simulink model "SILexample"  (R2024a)
settings: Solver=ode8  StartTime=0.0  StopTime=inf  FixedStep=SampleTime  RelTol=1e-3
undefined symbols (not defined in the file or in its folder): Arm, CDDrone, CDval, contact, control, ddx, ddy, ddz, dx, dy, dz, fractalcoef, g, lastVh, m, m_to_mm, p, pitch, prop_inertia, q, R, r, ref_height, ref_lat, ref_lon, roll, rotorRPMMax, rotorTimeConst, SampleTime, tilt_speed, X, Y, yaw, Z
libraries: sharedutil x3, robotcorelib x2, simulink x2, library_GPSPackaging x1, library_IMUPackaging x1, library_PX4SITLSFunc x1, shared6dof x1, simulink_extras x1, matrix_library x1, aerolibatmos2 x1, sensorgpslib x1, mspsensorlib x1
(part 1 of 2)
settings Model: Creator=tommy  LastModifiedBy=tommy

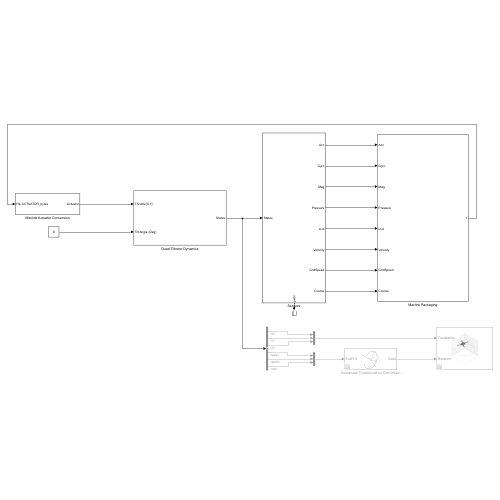
[thumbnail: Simulink's stored preview of the top-level diagram]
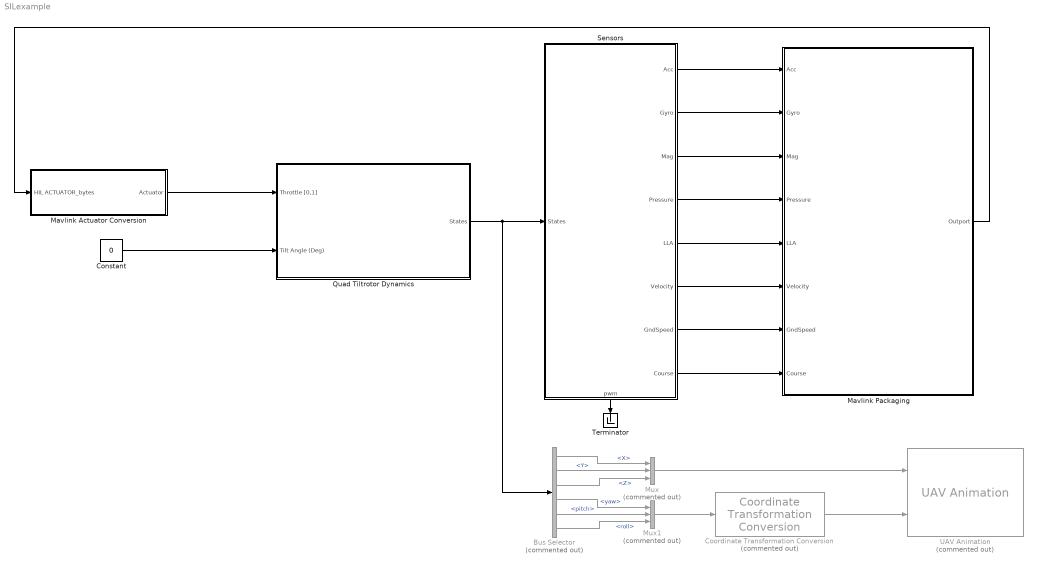
== system SILexample ==
  Bus Selector : BusSelector  Commented=on  OutputSignals=X,Y,Z,yaw,pitch,roll
  Constant : Constant  Value=0
  Coordinate Transformation Conversion : robotcorelib/Coordinate Transformation Conversion  Commented=on  InputRepresentation=Euler Angles  InputEulerSequence=ZYX  ShowTrVecInputPort=on  OutputRepresentation=Quaternion  OutputEulerSequence=ZYX  ShowTrVecOutputPort=on  SimulateUsing=Code generation
      settings: LibrarySourceBlock=uavutilslib/Coordinate Transformation Conversion
  Mavlink Actuator Conversion : Subsystem
  Mavlink Packaging : Subsystem
  Mux : Mux  Commented=on  Inputs=3
  Mux1 : Mux  Commented=on  Inputs=3
  Quad Tiltrotor Dynamics : Subsystem
  Sensors : Subsystem
      settings: PortSchema="{\"entries\":[{\"content\":{\"sides\":[{\"content\":{\"connectorIds\":[\"In1\"]},\"type\":\"ConnectorPlacement.EquallySpacedRectSide\",\"uuid\":\"4002fad5-cd2c-424c-b237-bc5c8c05716b\"},{\"content\":{\"connectorIds\":[\"Out1\",\"Out2\",\"Out3\",\"Out4\",\"Out5\",\"Out6\",\"Out7\",\"Out8\"],\"side\":\"RIGHT\"},\"type\":\"ConnectorPlacement.EquallySpacedRectSide\",\"uuid\":\"9eebcde2-0965-4c2d-bc23-958f112ae05f\"},{\"content\":{\"side\":\"TOP\"},\"type\":\"ConnectorPlacement.EquallySpacedRectSide\",\"uuid\":\"9f4a4643-69fe-47ac-ba33-df4cff119766\"},{\"content\":{\"connectorIds\":[\"Out9\"],\"side\":\"BOTTOM\"},\"type\":\"ConnectorPlacement.EquallySpacedRectSide\",\"uuid\":\"695c39dd-b607-453f-b052-38e279c7d42a\"}]},\"type\":\"ConnectorPlacement.EquallySpacedConnector\",\"uuid\":\"5d7ecaa3-fdec-470f-a1e1-b10a07dfac93\"}],\"packageUris\":[\"http://schema.mathworks.com/mf0/Connector/R2020b\"],\"version\":\"1.0\"}"
  Terminator : Terminator
  UAV Animation : uavutilslib/UAV Animation  Commented=on  UAVType=Multirotor  UAVSize=1  InertialZDirection=Down  SampleTime=0.04
  wires:
  Sensors/5(LLA) -> Mavlink Packaging/5(LLA)
  Sensors/1(Acc) -> Mavlink Packaging/1(Acc)
  Sensors/2(Gyro) -> Mavlink Packaging/2(Gyro)
  Sensors/3(Mag) -> Mavlink Packaging/3(Mag)
  Sensors/4(Pressure) -> Mavlink Packaging/4(Pressure)
  Sensors/6(Velocity) -> Mavlink Packaging/6(Velocity)
  Sensors/7(GndSpeed) -> Mavlink Packaging/7(GndSpeed)
  Sensors/8(Course) -> Mavlink Packaging/8(Course)
  Quad Tiltrotor Dynamics/1(States) -> Bus Selector/1, Sensors/1(States)
  Mavlink Actuator Conversion/1(Actuator) -> Quad Tiltrotor Dynamics/1(Throttle [0,1])
  Constant/1 -> Quad Tiltrotor Dynamics/2(Tilt Angle (Deg))
  Mux/1 -> UAV Animation/1
  Mux1/1 -> Coordinate Transformation Conversion/1
  Bus Selector/1 -> Mux/1  "<X>"
  Bus Selector/2 -> Mux/2  "<Y>"
  Bus Selector/3 -> Mux/3  "<Z>"
  Coordinate Transformation Conversion/1 -> UAV Animation/2
  Bus Selector/4 -> Mux1/1  "<yaw>"
  Bus Selector/5 -> Mux1/2  "<pitch>"
  Bus Selector/6 -> Mux1/3  "<roll>"
  Sensors/9(pwm) -> Terminator/1
  Mavlink Packaging/1(Outport) -> Mavlink Actuator Conversion/1(HIL ACTUATOR_bytes)

== system SILexample/Mavlink Actuator Conversion ==
  HIL ACTUATOR_bytes : Inport
  Data Type Conversion : DataTypeConversion  OutDataTypeStr=double  SaturateOnIntegerOverflow=off  RndMeth=Floor
  Rate Transition : RateTransition  OutPortSampleTime=SampleTime
  Saturation : Saturate  UpperLimit=1  LowerLimit=0
  Selector1 : Selector  InputPortWidth=16  IndexOptions=Index vector (dialog)  Indices=[1:4]  OutputSizes=1
  Actuator : Outport
  wires:
  Saturation/1 -> Actuator/1
  Data Type Conversion/1 -> Selector1/1
  Selector1/1 -> Saturation/1  "Controls"
  HIL ACTUATOR_bytes/1 -> Rate Transition/1
  Rate Transition/1 -> Data Type Conversion/1

== system SILexample/Mavlink Packaging ==
  Acc : Inport
  Gyro : Inport  Port=2
  Mag : Inport  Port=3
  Pressure : Inport  Port=4
  LLA : Inport  Port=5
  Velocity : Inport  Port=6
  GndSpeed : Inport  Port=7
  Course : Inport  Port=8
  GPSPackaging : library_GPSPackaging/GPSPackaging
  IMUPackaging : library_IMUPackaging/IMUPackaging
  PX4SITLSFunc : library_PX4SITLSFunc/PX4SITLSFunc
  Outport : Outport
  wires:
  Acc/1 -> IMUPackaging/1
  PX4SITLSFunc/1 -> Outport/1
  IMUPackaging/1 -> PX4SITLSFunc/1
  Gyro/1 -> IMUPackaging/2
  Mag/1 -> IMUPackaging/3
  Pressure/1 -> IMUPackaging/4
  LLA/1 -> GPSPackaging/1
  Velocity/1 -> GPSPackaging/2
  GndSpeed/1 -> GPSPackaging/3
  Course/1 -> GPSPackaging/4
  GPSPackaging/1 -> PX4SITLSFunc/2

== system SILexample/Quad Tiltrotor Dynamics ==
  note: Goals for this model : A novel vortex ring state escape mechanism for a quad tilt-rotor vehicle.
      |
      | 1. accurately portray thrust forces in a quad-tilt rotor vehicle in an in-place descent to design a controller for
      | - curve fits from CFD for descent in both non tilted and tilted configurations
      |
      | 2. simple transition model since horizontal forces and torques cancel out in both configurations
      | - transition interpolates forces between non tilted and tilted curves (based on angle)
      |
      | 3. simple model for torques since this research focuses more on in-place descents and less on attitude control
      | - torque model based on simple aerodynamics, e.g., assumption of constant Cd
  note: Note:
      |
      | DCM_be converts a vector written in earth frame to body frame
      | Abe is acceleration of body written in body frame, but measured relative to earth.
      | To get acceleration of body written in earth frame (NED fixed on takeoff location), we need to convert the frame.
      | IMU block's angular velocity and acceleration inputs are written in earth frame (NED)
  Throttle [0,1] : Inport
  Tilt Angle (Deg) : Inport  Port=2
  6DOF (Quaternion) : shared6dof/6DOF (Euler Angles)  units=Metric (MKS)  mtype=Fixed  rep=Quaternion  xme_0=init.posNED  Vm_0=init.vb  eul_0=init.euler  pm_0=init.angRates  mass_0=m  mass_e=0.5  mass_f=2.0  inertia=inertia  inertia_e=eye(3)  inertia_f=2*eye(3)  k_quat=1  vre_flag=on  abi_flag=on  aMode=0  xme_statename=''  Vm_statename=''  eul_statename=''  quat_statename=''  pm_statename=''  mass_statename=''
      settings: LibrarySourceBlock=aerolib6dof2/6DOF (Quaternion)
  Airframe : Subsystem
      mask Display: image('PX4-Quad-X-Motor-Configuration-33.png', [5,0,0,0,80,50]);
  Motor Model : Subsystem
  Rate Transition : RateTransition  OutPortSampleTime=SampleTime
  States Bus : Subsystem
  Terminator : Terminator
  Terminator1 : Terminator
  States : Outport
  wires:
  States Bus/1(States) -> Rate Transition/1
  Rate Transition/1 -> States/1
  6DOF (Quaternion)/7 -> Terminator/1
  6DOF (Quaternion)/4 -> Airframe/4(DCMbe), States Bus/4(DCMbe)
  6DOF (Quaternion)/6 -> Airframe/6(Wb), States Bus/5(Wb)
  Airframe/1(F_cg) -> 6DOF (Quaternion)/1
  6DOF (Quaternion)/2 -> States Bus/2(Xe), Airframe/5(Xe)
  Airframe/2(M_cg) -> 6DOF (Quaternion)/2
  6DOF (Quaternion)/9 -> States Bus/6(acc_lnav)
  6DOF (Quaternion)/5 -> Airframe/3(Vb)
  6DOF (Quaternion)/8 -> Terminator1/1
  6DOF (Quaternion)/3 -> Airframe/7(rpy), States Bus/3(rpy)
  6DOF (Quaternion)/1 -> States Bus/1(Ve)
  Tilt Angle (Deg)/1 -> Airframe/2(Tilt Angle (Deg))
  Throttle [0,1]/1 -> Motor Model/1(Throttle)
  Motor Model/1(RPM) -> Airframe/1(rpm)

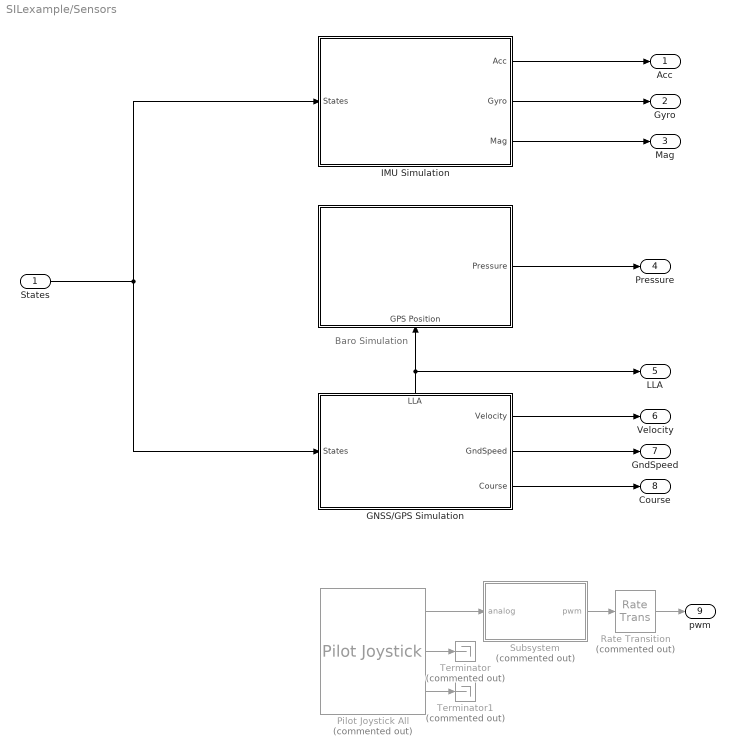
== system SILexample/Sensors ==
  note: Baro Simulation
  States : Inport
  " " : Subsystem
      settings: PortSchema="{\"entries\":[{\"content\":{\"sides\":[{\"content\":{\"connectorIds\":[]},\"type\":\"ConnectorPlacement.EquallySpacedRectSide\",\"uuid\":\"7ecc8b21-8f8f-4144-826a-6b68e30dbf7d\"},{\"content\":{\"connectorIds\":[\"Out1\"],\"side\":\"RIGHT\"},\"type\":\"ConnectorPlacement.EquallySpacedRectSide\",\"uuid\":\"81a1dd55-8330-4386-9921-36c0eb60d526\"},{\"content\":{\"connectorIds\":[],\"side\":\"TOP\"},\"type\":\"ConnectorPlacement.EquallySpacedRectSide\",\"uuid\":\"b99caff5-b40d-407d-b30e-35210c1aee1d\"},{\"content\":{\"connectorIds\":[\"In1\"],\"side\":\"BOTTOM\"},\"type\":\"ConnectorPlacement.EquallySpacedRectSide\",\"uuid\":\"18bfda3d-4fab-4e61-9ebc-e384e51de306\"}]},\"type\":\"ConnectorPlacement.EquallySpacedConnector\",\"uuid\":\"17ab4e96-b761-4c62-a0bb-ab626dac3eaa\"}],\"packageUris\":[\"http://schema.mathworks.com/mf0/Connector/R2020b\"],\"version\":\"1.0\"}"
  GNSS/GPS Simulation : Subsystem
      settings: PortSchema="{\"entries\":[{\"content\":{\"sides\":[{\"content\":{\"connectorIds\":[\"In1\"]},\"type\":\"ConnectorPlacement.EquallySpacedRectSide\",\"uuid\":\"4934e8ff-5d4b-4e11-968d-c23bd62383a0\"},{\"content\":{\"connectorIds\":[\"Out1\",\"Out2\",\"Out3\"],\"side\":\"RIGHT\"},\"type\":\"ConnectorPlacement.EquallySpacedRectSide\",\"uuid\":\"9ec8bc0a-2d3c-4dca-835c-010ac29b6ebc\"},{\"content\":{\"connectorIds\":[\"Out4\"],\"side\":\"TOP\"},\"type\":\"ConnectorPlacement.EquallySpacedRectSide\",\"uuid\":\"04f09eb4-1bd9-450e-b951-47054bdd92ad\"}]},\"type\":\"ConnectorPlacement.EquallySpacedConnector\",\"uuid\":\"9a5920cf-a58d-4c98-839b-fbac94edbe7e\"}],\"packageUris\":[\"http://schema.mathworks.com/mf0/Connector/R2020b\"],\"version\":\"1.0\"}"
  IMU Simulation : Subsystem
  Pilot Joystick All : aerolibanimutils/Pilot Joystick  Commented=on  JoystickID=Joystick1  OutputConfiguration=AllOutputs  SampleTime=0.04
  Rate Transition : RateTransition  Commented=on  OutPortSampleTime=SampleTime
  Subsystem : Subsystem  Commented=on
  Terminator : Terminator  Commented=on
  Terminator1 : Terminator  Commented=on
  Acc : Outport
  Gyro : Outport  Port=2
  Mag : Outport  Port=3
  Pressure : Outport  Port=4
  LLA : Outport  Port=5
  Velocity : Outport  Port=6
  GndSpeed : Outport  Port=7
  Course : Outport  Port=8
  pwm : Outport  Port=9
  wires:
  IMU Simulation/3(Mag) -> Mag/1
  GNSS/GPS Simulation/4(LLA) -> LLA/1, " "/1(GPS Position)
  GNSS/GPS Simulation/2(GndSpeed) -> GndSpeed/1
  States/1 -> GNSS/GPS Simulation/1(States), IMU Simulation/1(States)
  IMU Simulation/2(Gyro) -> Gyro/1
  IMU Simulation/1(Acc) -> Acc/1
  GNSS/GPS Simulation/1(Velocity) -> Velocity/1
  GNSS/GPS Simulation/3(Course) -> Course/1
  " "/1(Pressure) -> Pressure/1
  Pilot Joystick All/1 -> Subsystem/1(analog)
  Pilot Joystick All/2 -> Terminator/1
  Pilot Joystick All/3 -> Terminator1/1
  Subsystem/1(pwm) -> Rate Transition/1
  Rate Transition/1 -> pwm/1

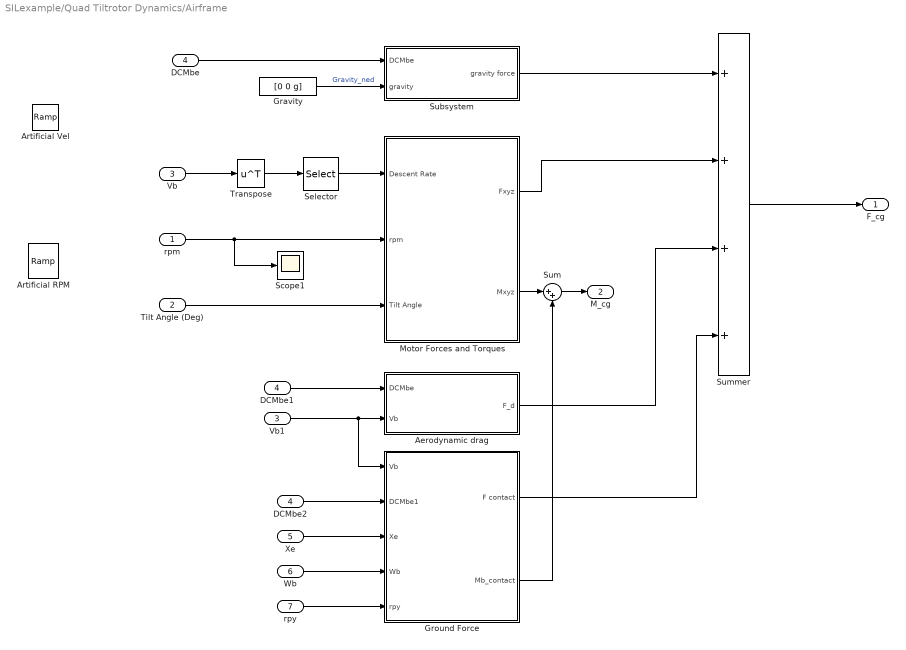
== system SILexample/Quad Tiltrotor Dynamics/Airframe ==
  rpm : Inport
  Tilt Angle (Deg) : Inport  Port=2
  Vb : Inport  Port=3
  DCMbe : Inport  Port=4
  Xe : Inport  Port=5
  Wb : Inport  Port=6
  rpy : Inport  Port=7
  Aerodynamic drag : Subsystem
  Artificial RPM : simulink/Sources/Ramp  slope=[0;-0;0;-0]  start=0  InitialOutput=[-3000; 3000; -2000; 2000]  VectorParams1D=off
  Artificial Vel : simulink/Sources/Ramp  slope=[0;0;0]  start=0  InitialOutput=[0;0;0]  VectorParams1D=off
  DCMbe1 : InportShadow  Port=4
  DCMbe2 : InportShadow  Port=4
  Gravity : Constant  Value=[0 0 g]
  Ground Force : Subsystem
  Motor Forces and Torques : Subsystem
  Scope1 : Scope
  Selector : Selector  InputPortWidth=3  IndexOptions=Index vector (dialog)  Indices=[3]  OutputSizes=1
  Subsystem : Subsystem
  Sum : Sum  Inputs=|++
  Summer : Sum  Inputs=++++
  Transpose : Math  Operator=transpose
  Vb1 : InportShadow  Port=3
  F_cg : Outport
  M_cg : Outport  Port=2
  wires:
  Subsystem/1(gravity force) -> Summer/1
  rpm/1 -> Scope1/1, Motor Forces and Torques/2(rpm)
  Motor Forces and Torques/1(Fxyz) -> Summer/2
  Gravity/1 -> Subsystem/2(gravity)  "Gravity_ned"
  DCMbe/1 -> Subsystem/1(DCMbe)
  Transpose/1 -> Selector/1
  Selector/1 -> Motor Forces and Torques/1(Descent Rate)
  Tilt Angle (Deg)/1 -> Motor Forces and Torques/3(Tilt Angle)
  Summer/1 -> F_cg/1
  Vb/1 -> Transpose/1
  DCMbe2/1 -> Ground Force/2(DCMbe1)
  Vb1/1 -> Ground Force/1(Vb), Aerodynamic drag/2(Vb)
  Xe/1 -> Ground Force/3(Xe)
  Aerodynamic drag/1(F_d) -> Summer/3
  Ground Force/1(F contact) -> Summer/4
  Ground Force/2(Mb_contact) -> Sum/2
  Motor Forces and Torques/2(Mxyz) -> Sum/1
  Sum/1 -> M_cg/1
  rpy/1 -> Ground Force/5(rpy)
  Wb/1 -> Ground Force/4(Wb)
  DCMbe1/1 -> Aerodynamic drag/1(DCMbe)

== system SILexample/Quad Tiltrotor Dynamics/Motor Model ==
  Throttle : Inport
  Demux : Demux
  Gain : Gain  Gain=[-1;-1;1;1]
  Mux : Mux
  Transfer Fcn{,2..4} (4 alike) : TransferFcn  Numerator=[rotorRPMMax]  Denominator=[rotorTimeConst 1]
  RPM : Outport
  wires:
  Mux/1 -> Gain/1
  Transfer Fcn/1 -> Mux/4
  Demux/4 -> Transfer Fcn/1
  Transfer Fcn3/1 -> Mux/2
  Transfer Fcn2/1 -> Mux/3
  Demux/1 -> Transfer Fcn4/1
  Demux/3 -> Transfer Fcn2/1
  Demux/2 -> Transfer Fcn3/1
  Transfer Fcn4/1 -> Mux/1
  Gain/1 -> RPM/1
  Throttle/1 -> Demux/1

== system SILexample/Quad Tiltrotor Dynamics/States Bus ==
  Ve : Inport
  Xe : Inport  Port=2
  rpy : Inport  Port=3
  DCMbe : Inport  Port=4
  Wb : Inport  Port=5
  acc_lnav : Inport  Port=6
  Bus Creator : BusCreator  Inputs=X,Y,Z,yaw,pitch,roll,dx,dy,dz,p,q,r,ddx,ddy,ddz
  Demux{,1..4} (5 alike) : Demux  Outputs=3
  Matrix Multiply : Product  Multiplication=Matrix(*)
  Matrix Multiply1 : Product  Multiplication=Matrix(*)
  Transpose : Math  Operator=transpose
  ypr : Selector  InputPortWidth=3  IndexOptions=Index vector (dialog)  Indices=[3 2 1]  OutputSizes=1
  States : Outport
  wires:
  Demux1/1 -> Bus Creator/1  "X"
  Demux1/2 -> Bus Creator/2  "Y"
  rpy/1 -> ypr/1
  Demux2/2 -> Bus Creator/5  "pitch"
  Demux3/2 -> Bus Creator/8  "dy"
  Demux2/3 -> Bus Creator/6  "roll"
  Ve/1 -> Demux3/1
  Demux2/1 -> Bus Creator/4  "yaw"
  Demux1/3 -> Bus Creator/3  "Z"
  Demux3/1 -> Bus Creator/7  "dx"
  Demux4/2 -> Bus Creator/11  "q"
  Demux3/3 -> Bus Creator/9  "dz"
  Demux4/3 -> Bus Creator/12  "r"
  Demux4/1 -> Bus Creator/10  "p"
  Bus Creator/1 -> States/1
  Xe/1 -> Demux1/1
  Demux/3 -> Bus Creator/15  "ddz"
  Demux/2 -> Bus Creator/14  "ddy"
  Demux/1 -> Bus Creator/13  "ddx"
  Matrix Multiply/1 -> Demux4/1
  DCMbe/1 -> Transpose/1
  Transpose/1 -> Matrix Multiply1/1, Matrix Multiply/1
  Wb/1 -> Matrix Multiply/2
  acc_lnav/1 -> Matrix Multiply1/2
  Matrix Multiply1/1 -> Demux/1
  ypr/1 -> Demux2/1

== system SILexample/Sensors/  ==
  GPS Position : Inport
  Extract Altitude : Selector  InputPortWidth=3  IndexOptions=Index vector (dialog)  Indices=[3]  OutputSizes=1
  Gain1 : Gain  Gain=1/m_to_mm
  Gain2 : Gain  Gain=m_to_mm
  Lapse Rate Model : aerolibatmos2/ISA Atmosphere Model  useExtended=off  action=Warning  custom=on  viscosityOut=off  g=9.80665  gamma=1.4  R=287.0531  L=0.0065  h_trop=11000  h_strat=20000  rho0=1.225  P0=101325  T0=288.15  h0=0  S=110.4  Tref=273.15  muref=1.716e-5
  Random Number1 : RandomNumber  Variance=10000  Seed=10  SampleTime=SampleTime
  Sum1 : Sum  Inputs=|++
  Terminator : Terminator
  Terminator1 : Terminator
  Terminator2 : Terminator
  Pressure : Outport
  wires:
  Lapse Rate Model/2 -> Terminator1/1
  Lapse Rate Model/4 -> Terminator2/1
  Lapse Rate Model/1 -> Terminator/1
  Lapse Rate Model/3 -> Pressure/1
  Sum1/1 -> Gain1/1
  Gain2/1 -> Sum1/1
  Extract Altitude/1 -> Gain2/1
  Gain1/1 -> Lapse Rate Model/1
  GPS Position/1 -> Extract Altitude/1
  Random Number1/1 -> Sum1/2  "Pressure_noise"

== system SILexample/Sensors/GNSS//GPS Simulation ==
  States : Inport
  Bus Selector : BusSelector  OutputSignals=dx,dy,dz  OutputAsBus=on
  Bus Selector1 : BusSelector  OutputSignals=X,Y,Z  OutputAsBus=on
  GPS : sensorgpslib/GPS  DispRefFrame=NED  PositionInputFormat=Local  ReferenceLocation=[ref_lat ref_lon ref_height]  HorizontalPositionAccuracy=0.01  VerticalPositionAccuracy=0.01  VelocityAccuracy=0.01  DecayFactor=0.99  SeedDouble=67  SimulateUsing=Interpreted execution
  Reshape1 : Reshape  OutputDimensionality=Row vector (2-D)
  Reshape3 : Reshape  OutputDimensionality=Row vector (2-D)
  Velocity : Outport
  GndSpeed : Outport  Port=2
  Course : Outport  Port=3
  LLA : Outport  Port=4
  wires:
  Reshape3/1 -> GPS/1
  GPS/1 -> LLA/1  "lla"
  Bus Selector1/1 -> Reshape3/1
  Bus Selector/1 -> Reshape1/1
  Reshape1/1 -> GPS/2
  GPS/2 -> Velocity/1
  States/1 -> Bus Selector/1, Bus Selector1/1
  GPS/3 -> GndSpeed/1
  GPS/4 -> Course/1

== system SILexample/Sensors/IMU Simulation ==
  note: Note:
      | we need accelerometer output)in A-G, but block outputs G-A.
  States : Inport
  Bus Selector1 : BusSelector  OutputSignals=p,q,r  OutputAsBus=on
  Bus Selector2 : BusSelector  OutputSignals=yaw,pitch,roll  OutputAsBus=on
  Bus Selector3 : BusSelector  OutputSignals=ddx,ddy,ddz  OutputAsBus=on
  Coordinate Transformation Conversion1 : robotcorelib/Coordinate Transformation Conversion  InputRepresentation=Euler Angles  InputEulerSequence=ZYX  ShowTrVecInputPort=on  OutputRepresentation=Quaternion  OutputEulerSequence=ZYX  ShowTrVecOutputPort=on  SimulateUsing=Interpreted execution
  Gain : Gain  Gain=-1
  IMU1 : mspsensorlib/IMU  DispRefFrame=NED  TemperaturePort=off  Temperature=25  MagneticFieldPort=off  MagneticFieldNED=[21.5 1.16 43.1]  MagneticFieldENU=[ -2.4169, 27.5550, 16.0849 ]  SeedDouble=87254  SimulateUsing=Interpreted execution  AccelParamsMeasurementRange=Inf  AccelParamsResolution=0  AccelParamsConstantBias=[ 0, 0, 0 ]  AccelParamsAxesMisalignment=[ 0, 0, 0 ]  AccelParamsNoiseDensity=0.0003  AccelParamsBiasInstability=[ 0, 0, 0 ]  AccelParamsBiasInstabilityNumerator=fractalcoef().Numerator  AccelParamsBiasInstabilityDenominator=fractalcoef().Denominator  AccelParamsRandomWalk=[ 0, 0, 0 ]  AccelParamsNoiseType=double-sided  AccelParamsTemperatureBias=[ 0, 0, 0 ]  AccelParamsTemperatureScaleFactor=[ 0, 0, 0 ]  GyroParamsMeasurementRange=Inf  GyroParamsResolution=0  GyroParamsConstantBias=[ 0, 0, 0 ]  GyroParamsAxesMisalignment=[ 0, 0, 0 ]  GyroParamsAccelerationBias=0.0001  GyroParamsNoiseDensity=0.01  GyroParamsBiasInstability=[ 0, 0, 0 ]  GyroParamsBiasInstabilityNumerator=fractalcoef().Numerator  GyroParamsBiasInstabilityDenominator=fractalcoef().Denominator  GyroParamsRandomWalk=[ 0, 0, 0 ]  GyroParamsNoiseType=double-sided  GyroParamsTemperatureBias=[ 0, 0, 0 ]  GyroParamsTemperatureScaleFactor=[ 0, 0, 0 ]  MagParamsMeasurementRange=Inf  MagParamsResolution=0  MagParamsConstantBias=[ 0, 0, 0 ]  MagParamsAxesMisalignment=[ 0, 0, 0 ]  MagParamsNoiseDensity=0.0001  MagParamsBiasInstability=[ 0, 0, 0 ]  MagParamsBiasInstabilityNumerator=fractalcoef().Numerator  MagParamsBiasInstabilityDenominator=fractalcoef().Denominator  MagParamsRandomWalk=[ 0, 0, 0 ]  MagParamsNoiseType=double-sided  MagParamsTemperatureBias=[ 0, 0, 0 ]  MagParamsTemperatureScaleFactor=[ 0, 0, 0 ]
  Reshape : Reshape  OutputDimensionality=Row vector (2-D)
  Reshape2 : Reshape  OutputDimensionality=Row vector (2-D)
  Reshape3 : Reshape  OutputDimensionality=Row vector (2-D)
  Acc : Outport
  Gyro : Outport  Port=2
  Mag : Outport  Port=3
  wires:
  Coordinate Transformation Conversion1/1 -> Reshape3/1
  Reshape3/1 -> IMU1/3
  IMU1/2 -> Gyro/1
  Reshape/1 -> IMU1/1
  Bus Selector3/1 -> Reshape/1
  IMU1/1 -> Gain/1
  Bus Selector1/1 -> Reshape2/1
  Bus Selector2/1 -> Coordinate Transformation Conversion1/1
  Reshape2/1 -> IMU1/2
  States/1 -> Bus Selector1/1, Bus Selector2/1, Bus Selector3/1
  Gain/1 -> Acc/1  "acc"
  IMU1/3 -> Mag/1

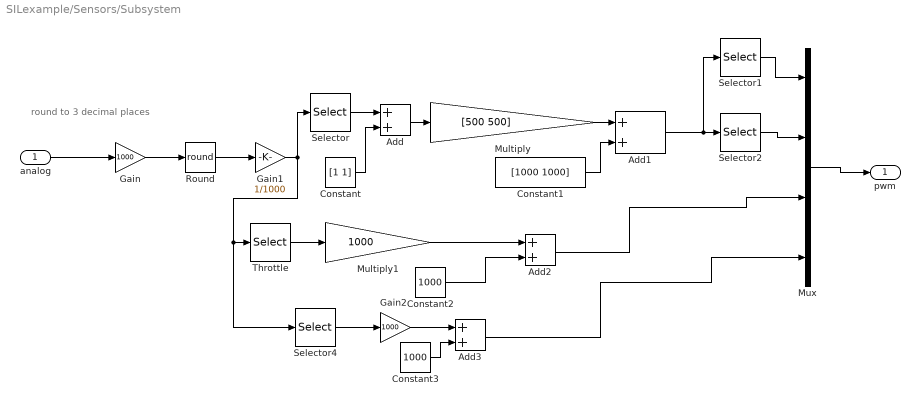
== system SILexample/Sensors/Subsystem ==
  note: round to 3 decimal places
  analog : Inport
  Add{,1..3} (4 alike) : Sum
  Constant : Constant  Value=[1 1]
  Constant1 : Constant  Value=[1000 1000]
  Constant2 : Constant  Value=1000
  Constant3 : Constant  Value=1000
  Gain : Gain  Gain=1000
  Gain1 : Gain  Gain=1/1000
  Gain2 : Gain  Gain=1000
  Multiply : Gain  Gain=[500 500]
  Multiply1 : Gain  Gain=1000
  Mux : Mux
  Round : Rounding  Operator=round
  Selector : Selector  InputPortWidth=6  IndexOptions=Index vector (dialog)  Indices=[1 2]  OutputSizes=1
  Selector1 : Selector  InputPortWidth=2  IndexOptions=Index vector (dialog)  Indices=[1]  OutputSizes=1
  Selector2 : Selector  InputPortWidth=2  IndexOptions=Index vector (dialog)  Indices=[2]  OutputSizes=1
  Selector4 : Selector  InputPortWidth=6  IndexOptions=Index vector (dialog)  Indices=[6]  OutputSizes=1
  Throttle : Selector  InputPortWidth=6  IndexOptions=Index vector (dialog)  Indices=[3]  OutputSizes=1
  pwm : Outport
  wires:
  Selector2/1 -> Mux/2
  Multiply/1 -> Add1/1
  Gain1/1 -> Selector4/1, Throttle/1, Selector/1
  Selector/1 -> Add/1
  Add1/1 -> Selector1/1, Selector2/1
  Gain/1 -> Round/1
  Constant/1 -> Add/2
  Constant2/1 -> Add2/2
  Add3/1 -> Mux/4
  Constant1/1 -> Add1/2
  Selector1/1 -> Mux/1
  analog/1 -> Gain/1
  Add/1 -> Multiply/1
  Round/1 -> Gain1/1
  Add2/1 -> Mux/3
  Throttle/1 -> Multiply1/1
  Multiply1/1 -> Add2/1
  Selector4/1 -> Gain2/1
  Constant3/1 -> Add3/2
  Gain2/1 -> Add3/1
  Mux/1 -> pwm/1

== system SILexample/Quad Tiltrotor Dynamics/Airframe/Aerodynamic drag ==
  DCMbe : Inport
  Vb : Inport  Port=2
  Add : Sum
  Constant : Constant  Value=[ 0 0 0]
  Constant1 : Constant  Value=CDDrone
  Display : Display
  Dot Product : DotProduct  OutDataTypeStr=Inherit: Inherit via internal rule
  Matrix Multiply : Product  Multiplication=Matrix(*)
  Product : Product  Inputs=3
  Saturation : Saturate  UpperLimit=inf  LowerLimit=0.0001
  Square Root : Sqrt
  gain : Gain  Gain=-1
  F_d : Outport
  wires:
  Saturation/1 -> Square Root/1
  Vb/1 -> gain/1
  Dot Product/1 -> Saturation/1
  Square Root/1 -> Product/1
  Constant1/1 -> Product/3
  DCMbe/1 -> Matrix Multiply/1
  Constant/1 -> Matrix Multiply/2
  gain/1 -> Add/2
  Matrix Multiply/1 -> Add/1
  Add/1 -> Dot Product/1, Dot Product/2, Product/2
  Product/1 -> Display/1, F_d/1

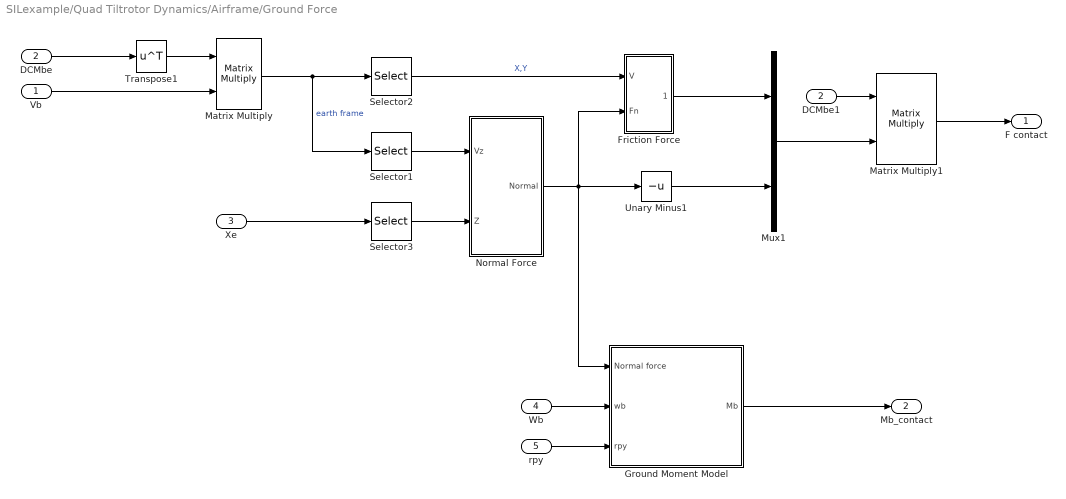
== system SILexample/Quad Tiltrotor Dynamics/Airframe/Ground Force ==
  Vb : Inport
  DCMbe1 : Inport  Port=2
  Xe : Inport  Port=3
  Wb : Inport  Port=4
  rpy : Inport  Port=5
  DCMbe : InportShadow  Port=2
  Friction Force : Subsystem
  Ground Moment Model : Subsystem
  Matrix Multiply : Product  Multiplication=Matrix(*)
  Matrix Multiply1 : Product  Multiplication=Matrix(*)
  Mux1 : Mux  Inputs=2
  Normal Force : Subsystem
  Selector1 : Selector  InputPortWidth=3  IndexOptions=Index vector (dialog)  Indices=[3]  OutputSizes=1
  Selector2 : Selector  InputPortWidth=3  IndexOptions=Index vector (dialog)  Indices=[1,2]  OutputSizes=1
  Selector3 : Selector  InputPortWidth=3  IndexOptions=Index vector (dialog)  Indices=[3]  OutputSizes=1
  Transpose1 : Math  Operator=transpose
  Unary Minus1 : UnaryMinus
  F contact : Outport
  Mb_contact : Outport  Port=2
  wires:
  Matrix Multiply1/1 -> F contact/1
  Friction Force/1(Friction) -> Mux1/1
  Xe/1 -> Selector3/1
  Vb/1 -> Matrix Multiply/2
  Selector3/1 -> Normal Force/2(Z)
  Matrix Multiply/1 -> Selector1/1, Selector2/1  "earth frame"
  Mux1/1 -> Matrix Multiply1/2
  Selector2/1 -> Friction Force/1(V)  "X,Y"
  Selector1/1 -> Normal Force/1(Vz)
  DCMbe1/1 -> Matrix Multiply1/1
  DCMbe/1 -> Transpose1/1
  Transpose1/1 -> Matrix Multiply/1
  Unary Minus1/1 -> Mux1/2
  Normal Force/1(Normal) -> Ground Moment Model/1(Normal force), Unary Minus1/1, Friction Force/2(Fn)
  Wb/1 -> Ground Moment Model/2(wb)
  rpy/1 -> Ground Moment Model/3(rpy)
  Ground Moment Model/1(Mb) -> Mb_contact/1

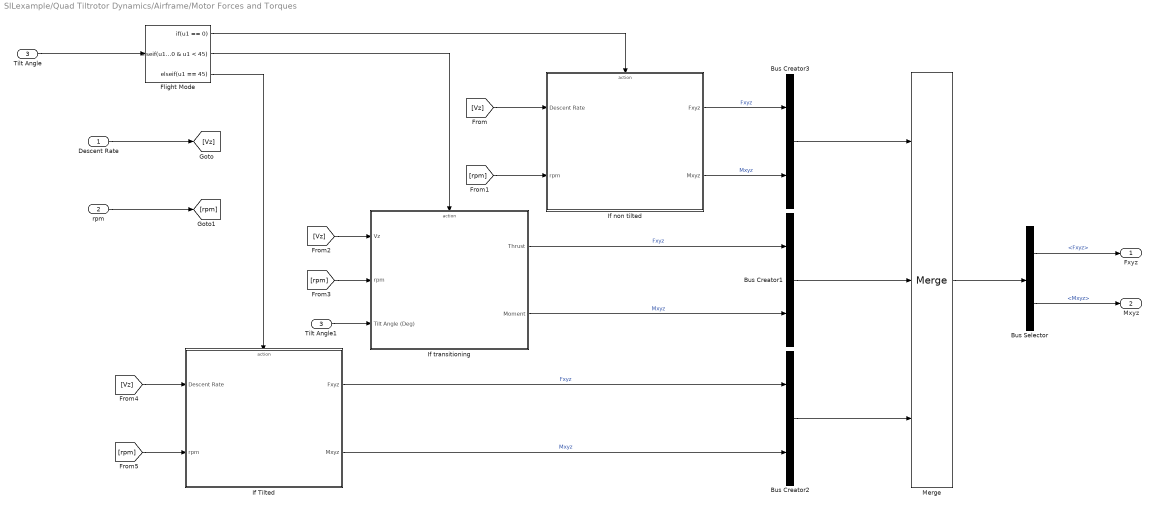
== system SILexample/Quad Tiltrotor Dynamics/Airframe/Motor Forces and Torques ==
  Descent Rate : Inport
  rpm : Inport  Port=2
  Tilt Angle : Inport  Port=3
  Bus Creator1 : BusCreator  Inputs=2
  Bus Creator2 : BusCreator  Inputs=2
  Bus Creator3 : BusCreator  Inputs=2
  Bus Selector : BusSelector  OutputSignals=Fxyz,Mxyz
  Flight Mode : If  IfExpression=u1 == 0  ElseIfExpressions=u1 > 0 & u1 < 45, u1 == 45  ShowElse=off
  If Tilted : Subsystem  TreatAsAtomicUnit=on
  If non tilted : Subsystem  TreatAsAtomicUnit=on
  If transitioning : Subsystem  TreatAsAtomicUnit=on
  Merge : Merge  Inputs=3  InitialOutput=[0]
  Tilt Angle1 : InportShadow  Port=3
  Fxyz : Outport
  Mxyz : Outport  Port=2
  wires:
  Flight Mode/3 -> If Tilted/Action
  Flight Mode/2 -> If transitioning/Action
  Flight Mode/1 -> If non tilted/Action
  Descent Rate/1 -> [Vz]
  rpm/1 -> [rpm]
  [Vz] -> If transitioning/1(Vz)
  [rpm] -> If transitioning/2(rpm)
  [Vz] -> If Tilted/1(Descent Rate)
  [rpm] -> If Tilted/2(rpm)
  If transitioning/1(Thrust) -> Bus Creator1/1  "Fxyz"
  If transitioning/2(Moment) -> Bus Creator1/2  "Mxyz"
  If Tilted/1(Fxyz) -> Bus Creator2/1  "Fxyz"
  If Tilted/2(Mxyz) -> Bus Creator2/2  "Mxyz"
  Bus Creator3/1 -> Merge/1
  Bus Creator1/1 -> Merge/2
  Merge/1 -> Bus Selector/1
  Bus Selector/1 -> Fxyz/1  "<Fxyz>"
  Bus Selector/2 -> Mxyz/1  "<Mxyz>"
  Bus Creator2/1 -> Merge/3
  If non tilted/1(Fxyz) -> Bus Creator3/1  "Fxyz"
  If non tilted/2(Mxyz) -> Bus Creator3/2  "Mxyz"
  [Vz] -> If non tilted/1(Descent Rate)
  [rpm] -> If non tilted/2(rpm)
  Tilt Angle1/1 -> If transitioning/3(Tilt Angle (Deg))
  Tilt Angle/1 -> Flight Mode/1

== system SILexample/Quad Tiltrotor Dynamics/Airframe/Subsystem ==
  DCMbe : Inport
  gravity : Inport  Port=2  Unit=m/s^2
  Gain1 : Gain  Gain=m
  Product : Product  Multiplication=Matrix(*)
  gravity force : Outport  Unit=N  VectorParamsAs1DForOutWhenUnconnected=off
  wires:
  gravity/1 -> Gain1/1
  Product/1 -> gravity force/1
  DCMbe/1 -> Product/1
  Gain1/1 -> Product/2  "gravity force NED"

== system SILexample/Quad Tiltrotor Dynamics/Airframe/Ground Force/Friction Force ==
  V : Inport
  Fn : Inport  Port=2
  Product : Product
  Saturation : Saturate  UpperLimit=contact.translation.maxFriction  LowerLimit=-contact.translation.maxFriction
  Soft Coulomb Friction : Subsystem
  Unary Minus : UnaryMinus
  Friction : Outport
  wires:
  Fn/1 -> Product/2
  Soft Coulomb Friction/1(Out1) -> Product/1
  Product/1 -> Unary Minus/1
  V/1 -> Soft Coulomb Friction/1(In1)
  Unary Minus/1 -> Saturation/1
  Saturation/1 -> Friction/1

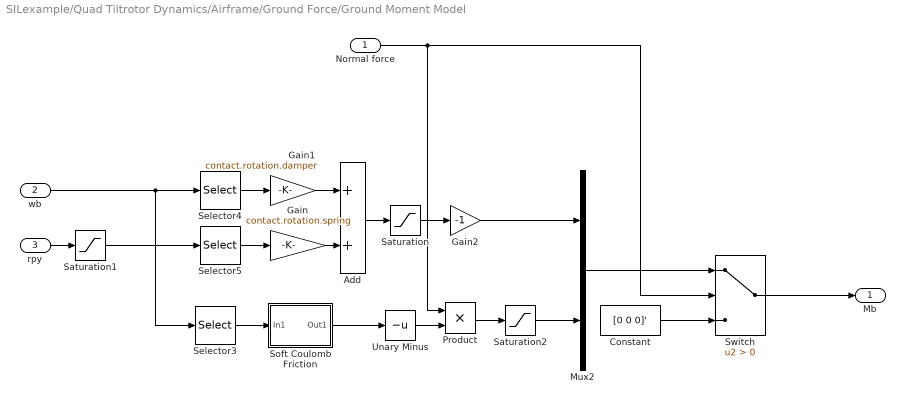
== system SILexample/Quad Tiltrotor Dynamics/Airframe/Ground Force/Ground Moment Model ==
  Normal force : Inport
  wb : Inport  Port=2
  rpy : Inport  Port=3
  Add : Sum
  Constant : Constant  Value=[0 0 0]'
  Gain : Gain  Gain=contact.rotation.spring
  Gain1 : Gain  Gain=contact.rotation.damper
  Gain2 : Gain  Gain=-1
  Mux2 : Mux  Inputs=2
  Product : Product
  Saturation : Saturate  UpperLimit=control.rotation.maxMoment  LowerLimit=-control.rotation.maxMoment
  Saturation1 : Saturate  UpperLimit=20*pi/180  LowerLimit=-20*pi/180
  Saturation2 : Saturate  UpperLimit=control.rotation.maxMoment  LowerLimit=-control.rotation.maxMoment
  Selector3 : Selector  InputPortWidth=3  IndexOptions=Index vector (dialog)  Indices=[3]  OutputSizes=1
  Selector4 : Selector  InputPortWidth=3  IndexOptions=Index vector (dialog)  Indices=[1, 2]  OutputSizes=1
  Selector5 : Selector  InputPortWidth=3  IndexOptions=Index vector (dialog)  Indices=[1, 2]  OutputSizes=1
  Soft Coulomb Friction : Subsystem
  Switch : Switch  Criteria=u2 > Threshold  SaturateOnIntegerOverflow=off  InputSameDT=off
  Unary Minus : UnaryMinus
  Mb : Outport
  wires:
  Gain2/1 -> Mux2/1
  Add/1 -> Saturation/1
  Gain/1 -> Add/2
  Saturation/1 -> Gain2/1
  Selector4/1 -> Gain1/1
  Gain1/1 -> Add/1
  Constant/1 -> Switch/3
  Selector5/1 -> Gain/1
  Switch/1 -> Mb/1
  Mux2/1 -> Switch/1
  Normal force/1 -> Product/1, Switch/2
  rpy/1 -> Saturation1/1
  Saturation1/1 -> Selector5/1
  wb/1 -> Selector4/1, Selector3/1
  Selector3/1 -> Soft Coulomb Friction/1(In1)
  Soft Coulomb Friction/1(Out1) -> Unary Minus/1
  Unary Minus/1 -> Product/2
  Product/1 -> Saturation2/1
  Saturation2/1 -> Mux2/2

== system SILexample/Quad Tiltrotor Dynamics/Airframe/Ground Force/Normal Force ==
  Vz : Inport
  Z : Inport  Port=2
  Add : Sum
  Constant : Constant  Value=0
  Damper Kp : Gain  Gain=-contact.translation.damper
  Saturation : Saturate  UpperLimit=contact.translation.maxNormal  LowerLimit=0
  Spring Kp : Gain  Gain=-contact.translation.spring
  Switch : Switch  Criteria=u2 > Threshold  SaturateOnIntegerOverflow=off  InputSameDT=off
  Unary Minus : UnaryMinus
  Unary Minus1 : UnaryMinus
  Normal : Outport
  wires:
  Constant/1 -> Switch/1
  Z/1 -> Unary Minus/1
  Switch/1 -> Saturation/1
  Damper Kp/1 -> Add/2
  Add/1 -> Switch/3
  Spring Kp/1 -> Add/1
  Vz/1 -> Unary Minus1/1
  Saturation/1 -> Normal/1
  Unary Minus/1 -> Spring Kp/1, Switch/2
  Unary Minus1/1 -> Damper Kp/1

== system SILexample/Quad Tiltrotor Dynamics/Airframe/Motor Forces and Torques/If Tilted ==
  Descent Rate : Inport
  rpm : Inport  Port=2
  Action Port : ActionPort  ActionPortLabel=elseif( u1 == 45)
  Constant : Constant  Value=1.225
  Constant1 : Constant  Value=Arm  VectorParams1D=off
  Multirotor Subsystem : Subsystem  TreatAsAtomicUnit=on
  Sum of Elements : Sum  Inputs=+  CollapseMode=Specified dimension  CollapseDim=2
  Sum of Elements1 : Sum  Inputs=+  CollapseMode=Specified dimension  CollapseDim=2
  Fxyz : Outport
  Mxyz : Outport  Port=2
  wires:
  Constant1/1 -> Multirotor Subsystem/4(Arm)
  Multirotor Subsystem/1(Thrust) -> Sum of Elements/1
  Sum of Elements1/1 -> Mxyz/1
  Descent Rate/1 -> Multirotor Subsystem/1(Descent Rate (+ve down))
  Constant/1 -> Multirotor Subsystem/2(rho)
  Sum of Elements/1 -> Fxyz/1
  rpm/1 -> Multirotor Subsystem/3(rpm)
  Multirotor Subsystem/2(Moment) -> Sum of Elements1/1

== system SILexample/Quad Tiltrotor Dynamics/Airframe/Motor Forces and Torques/If non tilted ==
  Descent Rate : Inport
  rpm : Inport  Port=2
  Action Port : ActionPort  ActionPortLabel=if(u1 == 0)
  Constant : Constant  Value=1.225
  Constant1 : Constant  Value=Arm  VectorParams1D=off
  Multirotor Subsystem : Subsystem  TreatAsAtomicUnit=on
  Sum of Elements : Sum  Inputs=+  CollapseMode=Specified dimension  CollapseDim=2
  Sum of Elements1 : Sum  Inputs=+  CollapseMode=Specified dimension  CollapseDim=2
  Fxyz : Outport
  Mxyz : Outport  Port=2
  wires:
  rpm/1 -> Multirotor Subsystem/3(rpm)
  Sum of Elements1/1 -> Mxyz/1
  Descent Rate/1 -> Multirotor Subsystem/1(Descent Rate (+ve down))
  Multirotor Subsystem/2(Moment) -> Sum of Elements1/1
  Constant/1 -> Multirotor Subsystem/2(rho)
  Constant1/1 -> Multirotor Subsystem/4(Arm)
  Multirotor Subsystem/1(Thrust) -> Sum of Elements/1
  Sum of Elements/1 -> Fxyz/1

== system SILexample/Quad Tiltrotor Dynamics/Airframe/Motor Forces and Torques/If transitioning ==
  Vz : Inport
  rpm : Inport  Port=2
  Tilt Angle (Deg) : Inport  Port=3
  Action Port : ActionPort  ActionPortLabel=elseif(u1 > 0 & u1 < 45)
  Constant1 : Constant  Value=Arm
  Degrees to Radians : simulink_extras/Transformations/Degrees to Radians
  Multirotor Subsystem : Subsystem  TreatAsAtomicUnit=on
  Sum of Elements : Sum  Inputs=+  CollapseMode=Specified dimension  CollapseDim=2
  Sum of Elements1 : Sum  Inputs=+  CollapseMode=Specified dimension  CollapseDim=2
  rho : Constant  Value=1.225
  Thrust : Outport
  Moment : Outport  Port=2
  wires:
  rpm/1 -> Multirotor Subsystem/3(rpm)
  rho/1 -> Multirotor Subsystem/2(rho)
  Vz/1 -> Multirotor Subsystem/1(Descent Rate (+ve down))
  Constant1/1 -> Multirotor Subsystem/4(Arm)
  Multirotor Subsystem/2(Moment) -> Sum of Elements1/1
  Multirotor Subsystem/1(Thrust) -> Sum of Elements/1
  Sum of Elements/1 -> Thrust/1
  Degrees to Radians/1 -> Multirotor Subsystem/5(Tilt Angle (rad))
  Tilt Angle (Deg)/1 -> Degrees to Radians/1
  Sum of Elements1/1 -> Moment/1

== system SILexample/Quad Tiltrotor Dynamics/Airframe/Ground Force/Friction Force/Soft Coulomb Friction ==
  note: Pennestrì, E., Rossi, V., Salvini, P. et al. Review and comparison of dry friction force models. Nonlinear Dyn 83, 1785–1801 (2016). https://doi.org/10.1007/s11071-015-2485-3
  In1 : Inport
  Tanh : Trigonometry  Operator=tanh
  friction coefficient : Gain  Gain=contact.translation.friction
  vd : Gain  Gain=1/contact.translation.vd
  Out1 : Outport
  wires:
  In1/1 -> vd/1
  vd/1 -> Tanh/1
  Tanh/1 -> friction coefficient/1
  friction coefficient/1 -> Out1/1

== system SILexample/Quad Tiltrotor Dynamics/Airframe/Ground Force/Ground Moment Model/Soft Coulomb Friction ==
  note: Pennestrì, E., Rossi, V., Salvini, P. et al. Review and comparison of dry friction force models. Nonlinear Dyn 83, 1785–1801 (2016). https://doi.org/10.1007/s11071-015-2485-3
  In1 : Inport
  Tanh : Trigonometry  Operator=tanh
  friction coefficient : Gain  Gain=control.rotation.friction
  vd : Gain  Gain=1/control.rotation.vd
  Out1 : Outport
  wires:
  In1/1 -> vd/1
  vd/1 -> Tanh/1
  Tanh/1 -> friction coefficient/1
  friction coefficient/1 -> Out1/1

== system SILexample/Quad Tiltrotor Dynamics/Airframe/Motor Forces and Torques/If Tilted/Multirotor Subsystem ==
  Descent Rate (+ve down) : Inport
  rho : Inport  Port=2
  rpm : Inport  Port=3  Partition=on  PartitionDimension=1  PartitionWidth=1  PartitionOffset=0
  Arm : Inport  Port=4  Partition=on  PartitionDimension=2  PartitionWidth=1  PartitionOffset=0
  For Each : ForEach  DisableCoverage=on
  Rotor Subsystem : Subsystem
  Thrust : Outport  ConcatenationDimension=2
  Moment : Outport  Port=2  ConcatenationDimension=2
  wires:
  Rotor Subsystem/4(Mxyz) -> Moment/1  "Moment"
  Arm/1 -> Rotor Subsystem/4(Arm)
  Descent Rate (+ve down)/1 -> Rotor Subsystem/1(Descent Rate (+ve down))
  rho/1 -> Rotor Subsystem/2(rho)
  Rotor Subsystem/3(Fxyz) -> Thrust/1  "Thrust"
  rpm/1 -> Rotor Subsystem/3(rpm)

== system SILexample/Quad Tiltrotor Dynamics/Airframe/Motor Forces and Torques/If non tilted/Multirotor Subsystem ==
  Descent Rate (+ve down) : Inport
  rho : Inport  Port=2
  rpm : Inport  Port=3  Partition=on  PartitionDimension=1  PartitionWidth=1  PartitionOffset=0
  Arm : Inport  Port=4  Partition=on  PartitionDimension=2  PartitionWidth=1  PartitionOffset=0
  For Each : ForEach  DisableCoverage=on
  Rotor Subsystem : Subsystem
  Thrust : Outport  ConcatenationDimension=2
  Moment : Outport  Port=2  ConcatenationDimension=2
  wires:
  Rotor Subsystem/4(Mxyz) -> Moment/1  "Moment"
  Arm/1 -> Rotor Subsystem/4(Arm)
  Descent Rate (+ve down)/1 -> Rotor Subsystem/1(Descent Rate (+ve down))
  rho/1 -> Rotor Subsystem/2(rho)
  Rotor Subsystem/3(Fxyz) -> Thrust/1  "Thrust"
  rpm/1 -> Rotor Subsystem/3(rpm)

== system SILexample/Quad Tiltrotor Dynamics/Airframe/Motor Forces and Torques/If transitioning/Multirotor Subsystem ==
  Descent Rate (+ve down) : Inport
  rho : Inport  Port=2
  rpm : Inport  Port=3  Partition=on  PartitionDimension=1  PartitionWidth=1  PartitionOffset=0
  Arm : Inport  Port=4  Partition=on  PartitionDimension=2  PartitionWidth=1  PartitionOffset=0
  Tilt Angle (rad) : Inport  Port=5
  For Each : ForEach  DisableCoverage=on
  Rotor Subsystem : Subsystem
  Thrust : Outport  ConcatenationDimension=2
  Moment : Outport  Port=2  ConcatenationDimension=2
  wires:
  Rotor Subsystem/4(Mxyz) -> Moment/1  "Moment"
  Arm/1 -> Rotor Subsystem/4(Arm)
  Descent Rate (+ve down)/1 -> Rotor Subsystem/1(Descent Rate (+ve down))
  rho/1 -> Rotor Subsystem/2(rho)
  Rotor Subsystem/3(Fxyz) -> Thrust/1  "Thrust"
  rpm/1 -> Rotor Subsystem/3(rpm)
  Tilt Angle (rad)/1 -> Rotor Subsystem/5(Tilt Angle (rad))

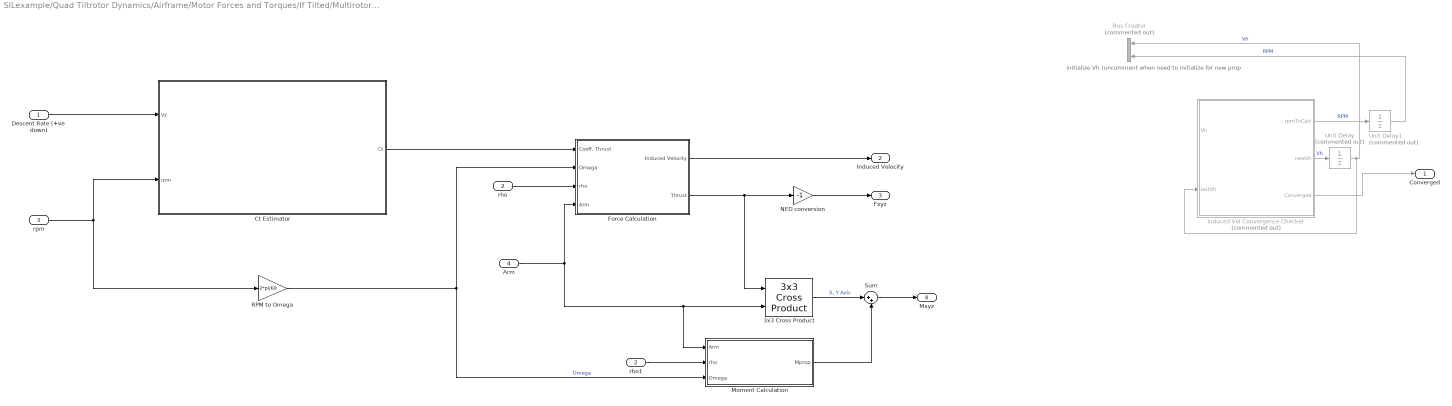
== system SILexample/Quad Tiltrotor Dynamics/Airframe/Motor Forces and Torques/If Tilted/Multirotor Subsystem/Rotor Subsystem ==
  note: initialize Vh (uncomment when need to initialize for new prop
  Descent Rate (+ve down) : Inport
  rho : Inport  Port=2
  rpm : Inport  Port=3
  Arm : Inport  Port=4
  3x3 Cross Product : sharedutil/3x3 Cross Product  aMode=aMode
      settings: LibrarySourceBlock=aerolibutil/3x3 Cross Product
  Bus Creator : BusCreator  Commented=on  Inputs=2
  Ct Estimator : Subsystem
  Force Calculation : Subsystem
  Induced Vel Convergence Checker : MATLAB Function  Commented=on  TreatAsAtomicUnit=on  mask{VhInit=4.7, ConvThresh=1e-4}
      mask prompts: VhInit "Initial Vh Guess"; ConvThresh "Convergence Threshold"
  Moment Calculation : Subsystem
  NED conversion : Gain  Gain=-1
  RPM to Omega : Gain  Gain=2*pi/60
  Sum : Sum  Inputs=|++
  Unit Delay : UnitDelay  Commented=on  InitialCondition=lastVh  SampleTime=0.001  HasFrameUpgradeWarning=on
  Unit Delay1 : UnitDelay  Commented=on  InitialCondition=1  SampleTime=0.001  HasFrameUpgradeWarning=on
  rho1 : InportShadow  Port=2
  Converged : Outport
  Induced Velocity : Outport  Port=2
  Fxyz : Outport  Port=3
  Mxyz : Outport  Port=4
  wires:
  Unit Delay/1 -> Bus Creator/1, Induced Vel Convergence Checker/2(lastVh)  "Vh"
  Induced Vel Convergence Checker/3(Converged) -> Converged/1
  RPM to Omega/1 -> Moment Calculation/3(Omega), Force Calculation/2(Omega)  "Omega"
  rho/1 -> Force Calculation/3(rho)
  Induced Vel Convergence Checker/2(newVh) -> Unit Delay/1  "Vh"
  rpm/1 -> Ct Estimator/2(rpm), RPM to Omega/1
  Unit Delay1/1 -> Bus Creator/2  "RPM"
  Induced Vel Convergence Checker/1(rpmToCalc) -> Unit Delay1/1  "RPM"
  Force Calculation/1(Induced Velocity) -> Induced Velocity/1
  Force Calculation/2(Thrust) -> NED conversion/1, 3x3 Cross Product/1
  3x3 Cross Product/1 -> Sum/1  "X, Y Axis"
  rho1/1 -> Moment Calculation/2(rho)
  Arm/1 -> Force Calculation/4(Arm), 3x3 Cross Product/2, Moment Calculation/1(Arm)
  Moment Calculation/1(Mprop) -> Sum/2
  Sum/1 -> Mxyz/1
  NED conversion/1 -> Fxyz/1
  Descent Rate (+ve down)/1 -> Ct Estimator/1(Vz)
  Ct Estimator/1(Ct) -> Force Calculation/1(Coeff. Thrust)

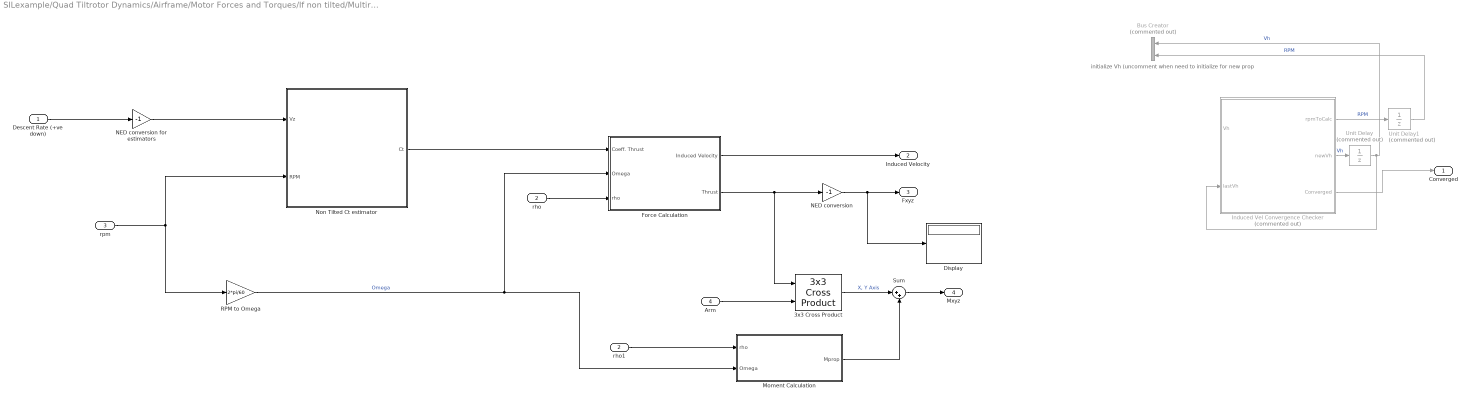
== system SILexample/Quad Tiltrotor Dynamics/Airframe/Motor Forces and Torques/If non tilted/Multirotor Subsystem/Rotor Subsystem ==
  note: initialize Vh (uncomment when need to initialize for new prop
  Descent Rate (+ve down) : Inport
  rho : Inport  Port=2
  rpm : Inport  Port=3
  Arm : Inport  Port=4
  3x3 Cross Product : sharedutil/3x3 Cross Product  aMode=aMode
      settings: LibrarySourceBlock=aerolibutil/3x3 Cross Product
  Bus Creator : BusCreator  Commented=on  Inputs=2
  Display : Display
  Force Calculation : Subsystem
  Induced Vel Convergence Checker : MATLAB Function  Commented=on  TreatAsAtomicUnit=on  mask{VhInit=4.7, ConvThresh=1e-4}
      mask prompts: VhInit "Initial Vh Guess"; ConvThresh "Convergence Threshold"
  Moment Calculation : Subsystem
  NED conversion : Gain  Gain=-1
  NED conversion for estimators : Gain  Gain=-1
  Non Tilted Ct estimator : Subsystem
  RPM to Omega : Gain  Gain=2*pi/60
  Sum : Sum  Inputs=|++
  Unit Delay : UnitDelay  Commented=on  InitialCondition=lastVh  SampleTime=0.001  HasFrameUpgradeWarning=on
  Unit Delay1 : UnitDelay  Commented=on  InitialCondition=1  SampleTime=0.001  HasFrameUpgradeWarning=on
  rho1 : InportShadow  Port=2
  Converged : Outport
  Induced Velocity : Outport  Port=2
  Fxyz : Outport  Port=3
  Mxyz : Outport  Port=4
  wires:
  Unit Delay/1 -> Bus Creator/1, Induced Vel Convergence Checker/2(lastVh)  "Vh"
  Induced Vel Convergence Checker/3(Converged) -> Converged/1
  RPM to Omega/1 -> Force Calculation/2(Omega), Moment Calculation/2(Omega)  "Omega"
  rho/1 -> Force Calculation/3(rho)
  Induced Vel Convergence Checker/2(newVh) -> Unit Delay/1  "Vh"
  rpm/1 -> Non Tilted Ct estimator/2(RPM), RPM to Omega/1
  Descent Rate (+ve down)/1 -> NED conversion for estimators/1
  Unit Delay1/1 -> Bus Creator/2  "RPM"
  Induced Vel Convergence Checker/1(rpmToCalc) -> Unit Delay1/1  "RPM"
  Force Calculation/1(Induced Velocity) -> Induced Velocity/1
  Force Calculation/2(Thrust) -> NED conversion/1, 3x3 Cross Product/1
  3x3 Cross Product/1 -> Sum/1  "X, Y Axis"
  rho1/1 -> Moment Calculation/1(rho)
  Arm/1 -> 3x3 Cross Product/2
  Moment Calculation/1(Mprop) -> Sum/2
  Sum/1 -> Mxyz/1
  NED conversion/1 -> Display/1, Fxyz/1
  NED conversion for estimators/1 -> Non Tilted Ct estimator/1(Vz)
  Non Tilted Ct estimator/1(Ct) -> Force Calculation/1(Coeff. Thrust)

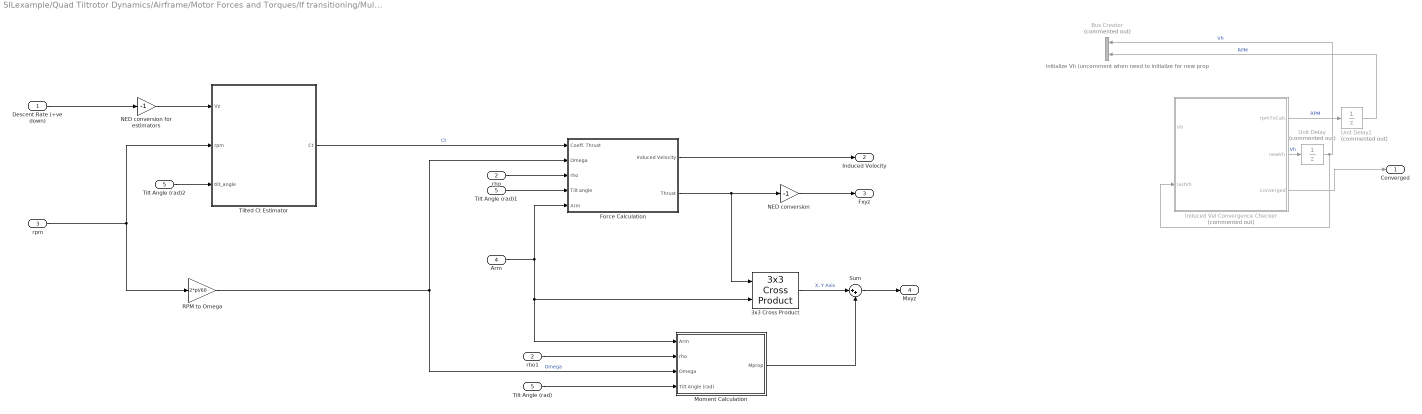
== system SILexample/Quad Tiltrotor Dynamics/Airframe/Motor Forces and Torques/If transitioning/Multirotor Subsystem/Rotor Subsystem ==
  note: initialize Vh (uncomment when need to initialize for new prop
  Descent Rate (+ve down) : Inport
  rho : Inport  Port=2
  rpm : Inport  Port=3
  Arm : Inport  Port=4
  Tilt Angle (rad) : Inport  Port=5
  3x3 Cross Product : sharedutil/3x3 Cross Product  aMode=aMode
      settings: LibrarySourceBlock=aerolibutil/3x3 Cross Product
  Bus Creator : BusCreator  Commented=on  Inputs=2
  Force Calculation : Subsystem
  Induced Vel Convergence Checker : MATLAB Function  Commented=on  TreatAsAtomicUnit=on  mask{VhInit=4.7, ConvThresh=1e-4}
      mask prompts: VhInit "Initial Vh Guess"; ConvThresh "Convergence Threshold"
  Moment Calculation : Subsystem
  NED conversion : Gain  Gain=-1
  NED conversion for estimators : Gain  Gain=-1
  RPM to Omega : Gain  Gain=2*pi/60
  Sum : Sum  Inputs=|++
  Tilt Angle (rad)1 : InportShadow  Port=5
  Tilt Angle (rad)2 : InportShadow  Port=5
  Tilted Ct Estimator : Subsystem
  Unit Delay : UnitDelay  Commented=on  InitialCondition=lastVh  SampleTime=0.001  HasFrameUpgradeWarning=on
  Unit Delay1 : UnitDelay  Commented=on  InitialCondition=1  SampleTime=0.001  HasFrameUpgradeWarning=on
  rho1 : InportShadow  Port=2
  Converged : Outport
  Induced Velocity : Outport  Port=2
  Fxyz : Outport  Port=3
  Mxyz : Outport  Port=4
  wires:
  Tilted Ct Estimator/1(Ct) -> Force Calculation/1(Coeff. Thrust)  "Ct"
  Unit Delay/1 -> Bus Creator/1, Induced Vel Convergence Checker/2(lastVh)  "Vh"
  Induced Vel Convergence Checker/3(Converged) -> Converged/1
  RPM to Omega/1 -> Moment Calculation/3(Omega), Force Calculation/2(Omega)  "Omega"
  rho/1 -> Force Calculation/3(rho)
  Induced Vel Convergence Checker/2(newVh) -> Unit Delay/1  "Vh"
  rpm/1 -> RPM to Omega/1, Tilted Ct Estimator/2(rpm)
  Descent Rate (+ve down)/1 -> NED conversion for estimators/1
  Unit Delay1/1 -> Bus Creator/2  "RPM"
  Induced Vel Convergence Checker/1(rpmToCalc) -> Unit Delay1/1  "RPM"
  Force Calculation/1(Induced Velocity) -> Induced Velocity/1
  Force Calculation/2(Thrust) -> NED conversion/1, 3x3 Cross Product/1
  3x3 Cross Product/1 -> Sum/1  "X, Y Axis"
  rho1/1 -> Moment Calculation/2(rho)
  Arm/1 -> 3x3 Cross Product/2, Moment Calculation/1(Arm), Force Calculation/5(Arm)
  Moment Calculation/1(Mprop) -> Sum/2
  Sum/1 -> Mxyz/1
  NED conversion/1 -> Fxyz/1
  Tilt Angle (rad)/1 -> Moment Calculation/4(Tilt Angle (rad))
  Tilt Angle (rad)1/1 -> Force Calculation/4(Tilt angle)
  NED conversion for estimators/1 -> Tilted Ct Estimator/1(Vz)
  Tilt Angle (rad)2/1 -> Tilted Ct Estimator/3(tilt_angle)

== system SILexample/Quad Tiltrotor Dynamics/Airframe/Motor Forces and Torques/If Tilted/Multirotor Subsystem/Rotor Subsystem/Ct Estimator ==
  note: this Vh curve is derived from performing a convergence
      | on the thrust curve
  note: Ct and Ct/Ct0 estimators are derived from CFD data
  Vz : Inport
  rpm : Inport  Port=2
  Abs : Abs  SaturateOnIntegerOverflow=off
  Calculate Ct : Product  Inputs=**
  Ct/C0 State Switcher : Subsystem
  Ct/Ct0 Estimator : Polyval  Coefs=[-0.012716815691322, -0.022830541813396, 0.156313447084851, -0.031641009616291, 1.004637965110952]
  Ct0 estimator for RPM : Polyval  Coefs=[0.000000000012185, -0.000000274732884, 0.008305365728125]
  Divide1 : Product  Inputs=*/
  NED conversion for estimators : Gain  Gain=-1
  Vh Calculator : Polyval  Coefs=[-5.17622414362771e-09, 0.000822973507549008, 0.0232660553338375]
  Ct : Outport
  wires:
  Abs/1 -> Ct0 estimator for RPM/1, Vh Calculator/1
  Divide1/1 -> Ct/Ct0 Estimator/1, Ct/C0 State Switcher/1(" Vz/Vh")  "Vz/Vh"
  Vh Calculator/1 -> Divide1/2  "Vh"
  Ct0 estimator for RPM/1 -> Calculate Ct/2  "Ct0"
  NED conversion for estimators/1 -> Divide1/1
  Ct/Ct0 Estimator/1 -> Ct/C0 State Switcher/2(Ct/C0 Fit)  "Ct/C0 Fit"
  Ct/C0 State Switcher/1(Out1) -> Calculate Ct/1  "Ct/C0"
  rpm/1 -> Abs/1
  Vz/1 -> NED conversion for estimators/1
  Calculate Ct/1 -> Ct/1  "Ct"

== system SILexample/Quad Tiltrotor Dynamics/Airframe/Motor Forces and Torques/If Tilted/Multirotor Subsystem/Rotor Subsystem/Force Calculation ==
  Coeff. Thrust : Inport
  Omega : Inport  Port=2
  rho : Inport  Port=3
  Arm : Inport  Port=4
  Constant : Constant  Value=0
  Divide : Product  Inputs=**
  Fx Sign : Subsystem
  Gain : Gain  Gain=cos(pi/4)
  Gain1 : Gain  Gain=sin(pi/4)
  Induced Vel Calc : Subsystem
  Math Function3 : Math  Operator=square  SignedPower=on
  Mux : Mux  Inputs=3
  Product6 : Product  Inputs=3
  R3 : Gain  Gain=R*R*pi*R*R
  Induced Velocity : Outport
  Thrust : Outport  Port=2
  wires:
  Math Function3/1 -> R3/1
  Induced Vel Calc/1(Vh) -> Induced Velocity/1
  R3/1 -> Product6/2
  Omega/1 -> Math Function3/1
  Gain1/1 -> Mux/3  "Fz"
  Constant/1 -> Mux/2  "Fy"
  Divide/1 -> Gain/1
  Product6/1 -> Divide/2, Gain1/1, Induced Vel Calc/1(Thrust)  "Fx"
  Fx Sign/1(Xsign) -> Divide/1
  Arm/1 -> Fx Sign/1(Arm)
  Gain/1 -> Mux/1  "Fx"
  Mux/1 -> Thrust/1
  Coeff. Thrust/1 -> Product6/3
  rho/1 -> Product6/1

== system SILexample/Quad Tiltrotor Dynamics/Airframe/Motor Forces and Torques/If Tilted/Multirotor Subsystem/Rotor Subsystem/Moment Calculation ==
  note: $\text{Torque about }z\text{ axis for the }i\text{th motor}: \frac{-1}{\sqrt2}(b\omega^2 + I_M \dot{w}), \text{where } b = \rho C_D AR^3$
  note: Angular Acceleration Term - $I_m \dot{\omega}$
  Arm : Inport
  rho : Inport  Port=2
  Omega : Inport  Port=3
  Abs : Abs  SaturateOnIntegerOverflow=off
  Divide : Product  Inputs=**
  Matrix Multiply : Product
  Moment of Inertia (1/12 m (a^2 + b^2)) : Gain  Gain=prop_inertia
  Mx Sign : Subsystem
  Mxy : Constant  Value=[0]
  OmegaDot : Derivative
  Product7 : Product
  R4 : Gain  Gain=CDval*R*R*R*pi*R*R
  Sum : Sum  Inputs=|++
  Vector Concatenate3 : Concatenate  NumInputs=3
  X : Gain  Gain=-1/sqrt(2)
  Z : Gain  Gain=-1/sqrt(2)
  Mprop : Outport
  wires:
  Vector Concatenate3/1 -> Mprop/1
  Omega/1 -> Abs/1, OmegaDot/1, Matrix Multiply/1
  OmegaDot/1 -> Moment of Inertia (1/12 m (a^2 + b^2))/1  "OmegaDot"
  Sum/1 -> Z/1, Divide/2
  Product7/1 -> Sum/1
  Moment of Inertia (1/12 m (a^2 + b^2))/1 -> Sum/2
  Z/1 -> Vector Concatenate3/3
  Divide/1 -> X/1
  Mxy/1 -> Vector Concatenate3/2  "Y"
  X/1 -> Vector Concatenate3/1
  Arm/1 -> Mx Sign/1(Arm)
  Mx Sign/1(Xsign) -> Divide/1
  Matrix Multiply/1 -> R4/1
  Abs/1 -> Matrix Multiply/2
  rho/1 -> Product7/1
  R4/1 -> Product7/2

== system SILexample/Quad Tiltrotor Dynamics/Airframe/Motor Forces and Torques/If non tilted/Multirotor Subsystem/Rotor Subsystem/Force Calculation ==
  Coeff. Thrust : Inport
  Omega : Inport  Port=2
  rho : Inport  Port=3
  Constant : Constant  Value=[0;0]  VectorParams1D=off
  Induced Vel Calc : Subsystem
  Math Function3 : Math  Operator=square  SignedPower=on
  Product6 : Product  Inputs=3
  R3 : Gain  Gain=R*R*pi*R*R
  Vector Concatenate : Concatenate
  Induced Velocity : Outport
  Thrust : Outport  Port=2
  wires:
  Coeff. Thrust/1 -> Product6/1
  Math Function3/1 -> R3/1
  Induced Vel Calc/1(Vh) -> Induced Velocity/1
  R3/1 -> Product6/2
  rho/1 -> Product6/3
  Omega/1 -> Math Function3/1
  Product6/1 -> Vector Concatenate/2, Induced Vel Calc/1(Thrust)  "Fz"
  Vector Concatenate/1 -> Thrust/1
  Constant/1 -> Vector Concatenate/1

== system SILexample/Quad Tiltrotor Dynamics/Airframe/Motor Forces and Torques/If non tilted/Multirotor Subsystem/Rotor Subsystem/Moment Calculation ==
  note: $\text{Torque about }z\text{ axis for the }i\text{th motor}: \frac{-1}{\sqrt2}(b\omega^2 + I_M \dot{w}), \text{where } b = \rho C_D AR^3$
  note: Angular Acceleration Term - $I_m \dot{\omega}$
  rho : Inport
  Omega : Inport  Port=2
  Abs : Abs  SaturateOnIntegerOverflow=off
  Matrix Multiply : Product
  Moment of Inertia (1/12 m (a^2 + b^2)) : Gain  Gain=prop_inertia
  Mxy : Constant  Value=[0;0]  VectorParams1D=off
  OmegaDot : Derivative
  Product7 : Product
  R4 : Gain  Gain=CDval*R*R*R*pi*R*R
  Sum : Sum  Inputs=|++
  Vector Concatenate3 : Concatenate
  Z : Gain  Gain=-1/sqrt(2)
  Mprop : Outport
  wires:
  Vector Concatenate3/1 -> Mprop/1
  R4/1 -> Product7/2
  rho/1 -> Product7/1
  Omega/1 -> Abs/1, OmegaDot/1, Matrix Multiply/1
  OmegaDot/1 -> Moment of Inertia (1/12 m (a^2 + b^2))/1  "OmegaDot"
  Sum/1 -> Z/1
  Product7/1 -> Sum/1
  Moment of Inertia (1/12 m (a^2 + b^2))/1 -> Sum/2
  Z/1 -> Vector Concatenate3/2
  Matrix Multiply/1 -> R4/1
  Abs/1 -> Matrix Multiply/2
  Mxy/1 -> Vector Concatenate3/1  "XY"

== system SILexample/Quad Tiltrotor Dynamics/Airframe/Motor Forces and Torques/If non tilted/Multirotor Subsystem/Rotor Subsystem/Non Tilted Ct estimator ==
  Vz : Inport
  RPM : Inport  Port=2
  Abs : Abs  SaturateOnIntegerOverflow=off
  Calculate Ct : Product  Inputs=**
  Ct/C0 State Switcher : Subsystem
  Ct/Ct0 Non Tilted Estimator : Polyval  Coefs=[0.147117704259973, 0.135195473604728, -0.341999514591595, -0.246799876690693, 0.999678014049876]
  Ct0 estimator for RPM : Polyval  Coefs=[0.000000000012185, -0.000000274732884, 0.008305365728125]
  Divide1 : Product  Inputs=*/
  Vh Calculator : Polyval  Coefs=[-5.17622414362771e-09, 0.000822973507549008, 0.0232660553338375]
  Ct : Outport
  wires:
  Abs/1 -> Vh Calculator/1, Ct0 estimator for RPM/1
  Calculate Ct/1 -> Ct/1  "Ct"
  Divide1/1 -> Ct/Ct0 Non Tilted Estimator/1, Ct/C0 State Switcher/1(" Vz/Vh")  "Vz/Vh"
  RPM/1 -> Abs/1
  Vh Calculator/1 -> Divide1/2  "Vh"
  Ct0 estimator for RPM/1 -> Calculate Ct/2  "Ct0"
  Ct/Ct0 Non Tilted Estimator/1 -> Ct/C0 State Switcher/2(Ct/C0 Fit)  "Ct/C0 Fit"
  Vz/1 -> Divide1/1
  Ct/C0 State Switcher/1(Ct/Ct0) -> Calculate Ct/1
